simulink library "AVE_Library"  (R2025b)
settings: Solver=VariableStepAuto  StartTime=0.0  StopTime=10.0  RelTol=1e-3
undefined symbols (not defined in the file or in its folder): DiscIntNeverNeededParam
libraries: simulink x44, etargetslib x18, $bdroot x13, GenericTarget x2
(part 5 of 5)

== matlab function AVE_Library/Navigation/Sensor Preprocessing/Butterworth Filter/Butterworth Low Pass and Derivation/Subsystem/myzp2ss ==
  data: z input; a output; p input; b output; c output; d output; nozerosFlag parameter size=1
function [a,b,c,d] = myzp2ss(z,p,nozerosFlag)
%%
%ZP2SS  Zero-pole to state-space conversion.
%   [A,B,C,D] = ZP2SS(Z,P,K)  calculates a state-space representation:
%       .
%       x = Ax + Bu
%       y = Cx + Du
%
%   for a system given a set of pole locations in column vector P,
%   a matrix Z with the zero locations in as many columns as there are
%   outputs, and the gains for each numerator transfer function in
%   vector K.  The A,B,C,D matrices are returned in block diagonal
%   form.  
%
%   The poles and zeros must correspond to a proper system. If the poles
%   or zeros are complex, they must appear in complex conjugate pairs,
%   i.e., the corresponding transfer function must be real.
%     
%   See also SS2ZP, ZP2TF, TF2ZP, TF2SS, SS2TF.

%   Thanks to G.F. Franklin
%   Copyright 1984-2008 The MathWorks, Inc.
% [z,p,k,isSIMO] = parse_input(z,p,k);
     isSIMO=false;
% if isSIMO
%     % If it's multi-output, we can't use the nice algorithm
%     % that follows, so use the numerically unreliable method
%     % of going through polynomial form, and then return.
%     [num,den] = zp2tf(z,p,k); % Suppress compile-time diagnostics
%     [a,b,c,d] = tf2ss(num,den);
%     return
% end

% Strip infinities and throw away.
% p = p(isfinite(p));
% z = z(isfinite(z));

% Group into complex pairs
np = length(p);

if nozerosFlag
    nz=0;
else
    nz = length(z);
end
% try
%     % z and p should have real elements and exact complex conjugate pair.
%     z = cplxpair(z,0);
%     p = cplxpair(p,0);
% catch
%     % If fail, revert to use the old default tolerance.
%     % The use of tolerance in checking for real entries and conjugate pairs
%     % may result in misinterpretation for edge cases. Please review the
%     % process of how z and p are generated.
%     z = cplxpair(z,1e6*nz*norm(z)*eps + eps);
%     p = cplxpair(p,1e6*np*norm(p)*eps + eps);
% end

% Initialize state-space matrices for running series

% a=[]; 
a=zeros(np);

b=zeros(np,1); c=ones(1,np); d=1;
% initial=false;
vollbis=0;
% If odd number of poles AND zeros, convert the pole and zero
% at the end into state-space.
%   H(s) = (s-z1)/(s-p1) = (s + num(2)) / (s + den(2))
if rem(np,2) && rem(nz,2)
    a(1,1) = real(p(np));
    b(1,1) = 1;
    c(1,1) = real(p(np)) - real(z(nz));
    d = 1;
    np = np - 1;
    nz = nz - 1;
%     initial=true;
    vollbis=1;
end

% If odd number of poles only, convert the pole at the
% end into state-space.
%  H(s) = 1/(s-p1) = 1/(s + den(2)) 
if rem(np,2)
    a(1,1) = real(p(np));
    b(1,1) = 1;
    c(1,1) = 1;
    d = 0;
    np = np - 1;
%     initial=true;
    vollbis=1;
end 

% If odd number of zeros only, convert the zero at the
% end, along with a pole-pair into state-space.
%   H(s) = (s+num(2))/(s^2+den(2)s+den(3)) 
if rem(nz,2)
    num = real(poly(z(nz)));
    den = real(poly(p(np-1:np)));
    wn = sqrt(prod(abs(p(np-1:np))));
    if wn == 0, wn = 1; end
    t = diag([1 1/wn]); % Balancing transformation
    a(1:2,1:2) = t\[-den(2) -den(3); 1 0]*t;
    b(1:2,1) = t\[1; 0];
    c(1,1:2) = [1 num(2)]*t;
    d = 0;
    nz = nz - 1;
    np = np - 2;
%     initial=true;
    vollbis=2;
end
%%
% Now we have an even number of poles and zeros, although not 
% necessarily the same number - there may be more poles.
%   H(s) = (s^2+num(2)s+num(3))/(s^2+den(2)s+den(3))
% Loop through rest of pairs, connecting in series to build the model.
i = 1;
% if i < nz
% a(1,1)=a(1,1);
% b(1,1)=b(1,1);
% c(1,1)=c(1,1);
% end
    
while i < nz
    index = i:i+1;
    num = real(poly(z(index)));
    den = real(poly(p(index)));
    wn = sqrt(prod(abs(p(index))));
    if wn == 0, wn = 1; end
    t = diag([1 1/wn]); % Balancing transformation
    a1 = t\[-den(2) -den(3); 1 0]*t; % 2x2 matrix
    b1 = t\[1; 0];% 2x1 matrix
    c1 = [num(2)-den(2) num(3)-den(3)]*t; % 1x2 matrix
    d1 = 1;
    % [a,b,c,d] = series(a,b,c,d,a1,b1,c1,d1); 
    % Next lines perform series connection 
%     ma1 = size(a,1);
%     na2 = size(a1,2);
if vollbis==0
    a(1:2,1:2)=[ a1];
%     b = [b; b1*d];
    b(1:2,1) = [b1*d];
%     c = [d1*c c1];
    c(1,1:2) = [c1];
%     initial=true;
    vollbis=2;
else
%     a = [a zeros(ma1,na2); b1*c a1];
Einsetzung=[b1*c(1:vollbis) a1];
nSpalteEinsetz=size(Einsetzung,2);
    a(vollbis+1:vollbis+2,1:nSpalteEinsetz)=Einsetzung;
%     b = [b; b1*d];
    b(vollbis+1:vollbis+2,1) = [b1*d];
%     c = [d1*c c1];
    c(1,1:vollbis+2) = [d1*c(1,1:vollbis) c1];
    vollbis=vollbis+2;        
end
    
    d = d1*d;

    i = i + 2;
end

% Take care of any left over unmatched pole pairs.
%   H(s) = 1/(s^2+den(2)s+den(3))
while i < np
    den = real(poly(p(i:i+1)));
    wn = sqrt(prod(abs(p(i:i+1))));
    if wn == 0, wn = 1; end
    t = diag([1 1/wn]); % Balancing transformation
    a1 = t\[-den(2) -den(3); 1 0]*t;
    b1 = t\[1; 0];
    c1 = [0 1]*t;
    d1 = 0;
    % [a,b,c,d] = series(a,b,c,d,a1,b1,c1,d1);
    % Next lines perform series connection 
%     ma1 = size(a,1);
%     na2 = size(a1,2);
%     a = [a zeros(ma1,na2); b1*c a1];

if vollbis==0
    a(1:2,1:2)=[ a1];
%     b = [b; b1*d];
    b(1:2,1) = [b1*d];
%     c = [d1*c c1];
    c(1,1:2) = [c1];
    c(1,1:vollbis+2) = [d1*c(1,1:vollbis) c1];
%     initial=true;
    vollbis=2;
else
    Einsetzung=[b1*c(1:vollbis) a1];
    nSpalteEinsetz=size(Einsetzung,2);    
    a(vollbis+1:vollbis+2,1:nSpalteEinsetz)=Einsetzung;
%     b = [b; b1*d];
    b(vollbis+1:vollbis+2,1) = [b1*d];
%     c = [d1*c c1];
    c(1,1:vollbis+2) = [d1*c(1,1:vollbis) c1];
    vollbis=vollbis+2;
end
d = d1*d;
    i = i + 2;
end

% % Apply gain k:
% c = c*k;
% d = d*k;
% 
% maxC=max(abs(c));
% c=c/maxC;
% b=b*maxC;



end

== matlab function AVE_Library/Essential/Signal Logics/Time To Latest Event/CalculateTimeToLatestEvent ==
  data: event input; timeToLatestEvent output; t input
function timeToLatestEvent = CalculateTimeToLatestEvent(event, t)
    persistent tPrev;
    if(isempty(tPrev))
        tPrev = -Inf;
    end
    if(event)
        tPrev = t;
    end
    timeToLatestEvent = t - tPrev;
end

== matlab function AVE_Library/Essential/Signal Logics/Push Buttons To Toggle Switches/MATLAB Function ==
  data: riseEvent input boolean; output output boolean; resetEvent input boolean size=1
function output = EventStateHandler(riseEvent, resetEvent)
    % Internal state (initial value is false)
    persistent state;
    if(isempty(state)), state = false(size(riseEvent)); end

    % Switch state if there's a rise event
    for i = 1:numel(riseEvent)
        if(riseEvent(i))
            state(i) = ~state(i);
        end
    end

    % Overwrite state if there's a reset event
    if(resetEvent)
        state = false(size(riseEvent));
    end
    output = state;
end

== matlab function AVE_Library/Essential/Transformation/Transform Sensor Velocity PQR/MATLAB Function ==
  data: pSensor input; pBody output; qSensor input; rSensor input; R_b2s input; qBody output; rBody output
function [pBody, qBody, rBody] = VelocityPQR_Sensor2Body(pSensor, qSensor, rSensor, R_b2s)
    [pBody, qBody, rBody] = ave.TransformSensor2BodyVelocityPQR(pSensor, qSensor, rSensor, R_b2s);
end

== matlab function AVE_Library/Essential/Transformation/Transform Sensor Euler ZYX/MATLAB Function ==
  data: rollSensor input; rollBody output; pitchSensor input; yawSensor input; R_b2s input; pitchBody output; yawBody output
function [rollBody, pitchBody, yawBody]= EulerZYX_Sensor2Body(rollSensor, pitchSensor, yawSensor, R_b2s)
    [rollBody, pitchBody, yawBody] = ave.TransformSensor2BodyEulerZYX(rollSensor, pitchSensor, yawSensor, R_b2s);
end

== matlab function AVE_Library/Essential/Smoothstep/MATLAB Function ==
  data: edge0 input; y output; edge1 input; x input
function y = Smoothstep(edge0, edge1, x)
    y = ave.Smoothstep(edge0, edge1, x);
end

== matlab function AVE_Library/Essential/Replace Nonfinite/MATLAB Function ==
  data: u input; y output; value parameter size=1
function y = ReplaceNonfinite(u, value)
    y = u;
    y(~isfinite(y)) = value;
end

== matlab function AVE_Library/Essential/Replace NaN/MATLAB Function ==
  data: u input double; y output double; value parameter double size=1
function y = ReplaceNaN(u, value)
    y = u;
    y(isnan(y)) = value;
end

== matlab function AVE_Library/Essential/Transformation/LLA To NED Vector/MATLAB Function ==
  data: positionLLA input; NED output; originLLA input
function NED = LLA2NEDv(positionLLA, originLLA)
    NED = ave.LLA2NED(positionLLA, originLLA);
end

== matlab function AVE_Library/Essential/Equations of Motion/Kinematic 6DoF Geographic/MATLAB Function2 ==
  data: Cb2n output; accelerationGravityCoriolis output; pqr_ib output; velocityNED output; uvwpqr_eb input; positionLLA input; dotPositionLLA output; quaternionWXYZ input; dotQuaternionWXYZ output
function [Cb2n, accelerationGravityCoriolis, pqr_ib, velocityNED, dotPositionLLA, dotQuaternionWXYZ] = ODEGeographic(uvwpqr_eb, positionLLA, quaternionWXYZ)
    % Get WGS84 parameters
    a = 6378137.0;
    ee = 0.00669437999014132;
    s = sin(positionLLA(1));
    invRoot = 1.0 ./ sqrt(1 - ee * s .* s);
    Re = a .* invRoot;
    Rn = Re .* (1-ee) .* (invRoot.*invRoot);
    omegaEarth = 7.292115e-5;
    gravity = ave.GravityWGS84(positionLLA(1), positionLLA(2), positionLLA(3));

    % Current rotation-based matrices
    Cb2n = quat2rotm([quaternionWXYZ(1), quaternionWXYZ(2), quaternionWXYZ(3), quaternionWXYZ(4)]);
    Ow = [
          -quaternionWXYZ(2) -quaternionWXYZ(3) -quaternionWXYZ(4);
           quaternionWXYZ(1) -quaternionWXYZ(4)  quaternionWXYZ(3);
           quaternionWXYZ(4)  quaternionWXYZ(1) -quaternionWXYZ(2);
          -quaternionWXYZ(3)  quaternionWXYZ(2)  quaternionWXYZ(1)
         ];

    % Velocity from b-frame to n-frame
    velocityNED = Cb2n * [uvwpqr_eb(1); uvwpqr_eb(2); uvwpqr_eb(3)];

    % Set d/dt output
    dotPositionLLA = diag([1.0/(Rn + positionLLA(3)), 1.0/(cos(positionLLA(1)) * (Re + positionLLA(3))), -1.0]) * velocityNED;
    dotQuaternionWXYZ = 0.5 * Ow * [uvwpqr_eb(4); uvwpqr_eb(5); uvwpqr_eb(6)];

    % Add earth rotation and transport rate to pqr_eb to obtain pqr_ib
    veOverReAlt = velocityNED(2) / (Re + positionLLA(3));
    earthRotationAndTransportRateNFrame = [omegaEarth * cos(positionLLA(1)) + veOverReAlt; -velocityNED(1) / (Rn + positionLLA(3)); -omegaEarth * sin(positionLLA(1)) - tan(positionLLA(1)) * veOverReAlt];
    pqr_ib = (Cb2n' * earthRotationAndTransportRateNFrame) + [uvwpqr_eb(4); uvwpqr_eb(5); uvwpqr_eb(6)];

    % Earth-fixed acceleration due to gravity and coriolis
    w_ie = [omegaEarth * cos(positionLLA(1)); 0; -omegaEarth * sin(positionLLA(1))];
    w_en = [(velocityNED(2) / ((Re + positionLLA(3)))); -(velocityNED(1) / (Rn + positionLLA(3))); -(velocityNED(2) / (Re + positionLLA(3)))*tan(positionLLA(1))];
    coriolis = cross(2.0 * w_ie + w_en, velocityNED);
    accelerationGravityCoriolis = coriolis - [0.0; 0.0; gravity];
end

== matlab function AVE_Library/Essential/Equations of Motion/Kinematic 6DoF Geographic/MATLAB Function3 ==
  data: velocityNED input; cog output; sog output; aoa output
function [cog, sog, aoa] = MovementOverGround(velocityNED)
    sog = sqrt(velocityNED(1)*velocityNED(1) + velocityNED(2)*velocityNED(2));
    cog = atan2(velocityNED(2), velocityNED(1));
    aoa = atan2(velocityNED(3), sog);
end

== matlab function AVE_Library/Essential/Transformation/NED To LLA Vector/MATLAB Function ==
  data: positionNED input; positionLLA output; originLLA input
function positionLLA = fcn(positionNED, originLLA)
    positionLLA = ave.NED2LLA(positionNED, originLLA);
end

== matlab function AVE_Library/Control/Input Delay Compensation Design/calculate weight matrix stack ==
  data: A input double size=[dimX, dimX]; W output double size=[dimX, dimU*maxNumDelays]; B input double size=[dimX, dimU]; num_delay_steps input int32 size=1; maxNumDelays parameter int32 size=1; SampleTime parameter double size=1; dimU parameter int32 size=1; dimX parameter int32 size=1
function W = CalculateWeightMatrixStack(A, B, num_delay_steps, maxNumDelays, SampleTime, dimU, dimX)
    % CalculateWeightMatrixStack Computes the row-stacked weight matrices for input delay compensation.
    % The weight matrix stack has the following format:
    % 
    % +-----+-----+-----+-----+-----+-----+-----+
    % | W_1 | W_2 | ... | W_N |  0  | ... |  0  |
    % +-----+-----+-----+-----+-----+-----+-----+
    % 
    % A matrix block W_i relates to the delayed input u(t - i*Ts). It is calculated by
    % W_i = expm(-A*Ts*(N - i)) * B
    % 
    % For efficient calculation using recursive multiplication, the matrices are calculated starting
    % with W_N and propagating to the front of the stack (W_1). In that way, expm is only calculated once.

    % initialize the full stack matrix with zeros
    W = zeros(dimX, dimU * maxNumDelays);

    % compute the base matrix exponential for one sample time: M = exp(-A * Ts)
    M = expm(-A * SampleTime);
    
    % initialize M_i to track powers of M (M^i)
    M_i = eye(dimX);
    
    % fill stack starting from N-th matrix, iterating to front of matrix stack
    N = min(num_delay_steps, maxNumDelays);
    for i = N:int32(-1):int32(1)
        j0 = int32(1) + (i - int32(1)) * dimU;   % starting index of i-th weight matrix
        j1 = j0 + dimU - int32(1);               % ending index of i-th weight matrix
        
        % compute and store the i-th weight matrix: W_i = exp(-A * Ts * (N-i)) * B
        W(:, j0:j1) = M_i * B;

        % efficiently compute M^i using recursive multiplication
        M_i = M_i * M;
    end
end

== matlab function AVE_Library/Control/Input Delay Compensation/Calculate Compensation Term ==
  data: u_prev input double size=[dimU,1]; weightMatrixStack input double size=[dimX, dimU*maxNumDelays]; dimU parameter int32 size=1; dimX parameter int32 size=1; x output double size=[dimX,1]; maxNumDelays parameter int32 size=1; SampleTime parameter double size=1; reset input boolean size=1
function x = DelayCompensationTerm(u_prev, weightMatrixStack, dimU, dimX, maxNumDelays, SampleTime, reset)
    % Calculate reduction term for input delay compensation.
    % 
    % References
    % Kwon, W. and Pearson, A. (1980). Feedback stabilization of linear systems with delayed control. IEEE Transactions on Automatic Control, 25(2), 266–269. doi:10.1109/TAC.1980.1102288.
    % 
    % INPUT
    % u_prev ... The previous input value (to be stored in a buffer containing delayed inputs)
    % weightMatrixStack ... Row-Stack of weight matrices [W1, W2, ..., Wn], each of them containing exp(-A(theta*h))*B1, see original paper.
    % reset ... Reset the buffer to zero.
    % 
    % PARAMETER
    % dimU ... Dimension of control input.
    % dimX ... Dimension of state vector.
    % maxNumDelays ... Maximum number of delayed control inputs to store.
    % SampleTime ... Discrete sampletime of the system.

    % persistent buffer and circular write index
    persistent u_buffer idx;
    if(isempty(u_buffer) || reset)
        u_buffer = zeros(dimU, maxNumDelays);
        idx = maxNumDelays;
    end

    % advance write index circularly and insert new value
    idx = mod(idx, maxNumDelays) + int32(1);
    u_buffer(:, idx) = u_prev;

    % apply compensation x = sum_k(W_k*u_k) * Ts
    x = zeros(dimX, 1);
    Wk = zeros(dimX, dimU);                                               % fixed-size local storage to make simulink happy
    for i = int32(1):maxNumDelays
        j0 = int32(1) + (i - int32(1)) * dimU;                            % starting index of i-th weight matrix
        j1 = j0 + dimU - int32(1);                                        % ending index of i-th weight matrix
        Wk(:,:) = weightMatrixStack(:,j0:j1);                             % assignment to fixed-sized storage to make simulink happy
        buf_idx = mod(idx - i + maxNumDelays, maxNumDelays) + int32(1);   % compute the correct buffer column for the i-th delay step
        x = x + Wk * u_buffer(:, buf_idx);
    end
    x = x * SampleTime;
end

== matlab function AVE_Library/Control/Aperiodic IT2 SISO Control with Integral Action and Input Delay/Controller Design/Controller Design ==
  data: k input; K output; kaw output; T1 input; T2 input; gamma input; mu input; beta input; Ai output; Bi output; h input
function [K, kaw, Ai, Bi] = ControllerDesign(k, T1, T2, gamma, mu, beta, h)
    e1 = exp(h / T1);
    e2 = exp(h / T2);
    b1 = k * (T1*(1.0 - e1) - T2*(1.0 - e2)) / (T1 - T2);
    b2 = k * (e1 - e2) / (T1 - T2);
    b3 = e2 / T2;
    b4 = k * (T1*T1*(1.0 - e1) - T2*T2*(1.0 - e2) + h*(T1 - T2)) / (T1 - T2);
    wc = gamma / max(T1, T2);
    mu2 = mu * mu;
    L1 = -wc;
    L2 = -mu * wc;
    L3 = -mu2 * wc;
    L4 = -mu2 * mu * wc;
    L1L2 = L1 * L2;
    L3L4 = L3 * L4;
    a0 = L1L2 * L3L4;
    a1 = -L1L2 * (L3 + L4) - L3L4 * (L1 + L2);
    a2 = L1 * (L2 + L3 + L4) + L2 * (L3 + L4) + L3L4;
    a3 = -L1 - L2 - L3 - L4;
    f0 = 1.0 / (T1 * T2);
    f1 = f0 * (T1 + T2);
    f2 = f1 * b1 + b2;
    f3 = f0 * (T1 * b2 + T2 * b3 * k);
    f4 = b3 / T1;
    f5 = f1 * b4 - b1;
    f6 = f0 * b1 + f3;
    f7 = f0 * b4 - f2;
    k4 = -a0 / f6;
    k1 = (a1 - f7 * k4) / f6;
    k3 = (f3*(a3 - f1 - b1*k1 - b4*k4) - b2*(a2 - f0 - f2*k1 - f5*k4)) / (f3 * b3 - b2 * f4);
    k2 = (a2 - f0 - f2*k1 - f5*k4 - f4*k3) / f3;

    K = [k1, k2, k3, k4];
    kaw = beta / abs(k4);
    Bi = [0; 0; 1/T2; 0];
    Ai = [0 1 0 0; 0 -1.0/T1 k/T1 0; 0 0 -1/T2 0; -1 0 0 0];
end

== matlab function AVE_Library/Essential/Transformation/LLA To NED/MATLAB Function ==
  data: lat input; N output; lon input; alt input; originLat input; originLon input; originAlt input; E output; D output
function [N, E, D] = LLA2NED(lat, lon, alt, originLat, originLon, originAlt)
    [N, E, D] = ave.LLA2NED(lat, lon, alt, originLat, originLon, originAlt);
end

== matlab function AVE_Library/Control/Aperiodic IT2 SISO Control with Integral Action and Input Delay/Controller Design/wrap to sampletime ==
  data: inputTimeDelay input double size=1; time_delay output double size=1; SampleTime parameter double size=1; num_delay_steps output int32 size=1; maxNumDelays parameter int32 size=1
function [time_delay, num_delay_steps] = WrapToSampletime(inputTimeDelay, SampleTime, maxNumDelays)
    tau = max(0.0, inputTimeDelay);
    num_delay_steps = min(int32(round(tau / SampleTime)), maxNumDelays);
    time_delay = double(num_delay_steps) * SampleTime;
end

== matlab function AVE_Library/Essential/Transformation/Quaternion To Euler ZYX/MATLAB Function ==
  data: q input; roll output; pitch output; yaw output
function [roll, pitch, yaw] = QuaternionToEulerZYX(q)
    eul = quat2eul([q(1), q(2), q(3), q(4)]);
    roll = ave.SymmetricalAngle(eul(3));
    pitch = ave.SymmetricalAngle(eul(2));
    yaw = ave.SymmetricalAngle(eul(1));
end

== matlab function AVE_Library/Essential/Transformation/Euler ZYX To Quaternion/MATLAB Function1 ==
  data: roll input; q output; pitch input; yaw input
function q = EulerZYXToQuaternion(roll, pitch, yaw)
    quat = eul2quat([yaw, pitch, roll]);
    q = [quat(1); quat(2); quat(3); quat(4)];
end

== matlab function AVE_Library/Essential/Transformation/NED To LLA/MATLAB Function ==
  data: N input; lat output; E input; D input; originLat input; originLon input; originAlt input; lon output; alt output
function [lat, lon, alt] = NED2LLA(N, E, D, originLat, originLon, originAlt)
    [lat, lon, alt] = ave.NED2LLA(N, E, D, originLat, originLon, originAlt);
end

== matlab function AVE_Library/Essential/Transformation/Quaternion To Rotation Matrix/MATLAB Function ==
  data: qb2n input; matCb2n output
function matCb2n = Cb2n(qb2n)
    q = [qb2n(1), qb2n(2), qb2n(3), qb2n(4)];
    matCb2n = quat2rotm(q);
end

== matlab function AVE_Library/Essential/Transformation/Transform Sensor Position LLA/MATLAB Function ==
  data: latSensor input; latBody output; lonSensor input; altSensor input; R_b2n input; r_b2s input; lonBody output; altBody output
function [latBody, lonBody, altBody] = PositionLLA_Sensor2Body(latSensor, lonSensor, altSensor, R_b2n, r_b2s)
    [latBody, lonBody, altBody] = ave.TransformSensor2BodyPositionLLA(latSensor, lonSensor, altSensor, R_b2n, r_b2s);
end
